simulink library "Teleop_lib"  (R2023b)
settings: Solver=VariableStepAuto  StartTime=0.0  StopTime=10.0  RelTol=1e-3
settings Model: Creator=FIRSTMentor  LastModifiedBy=ander

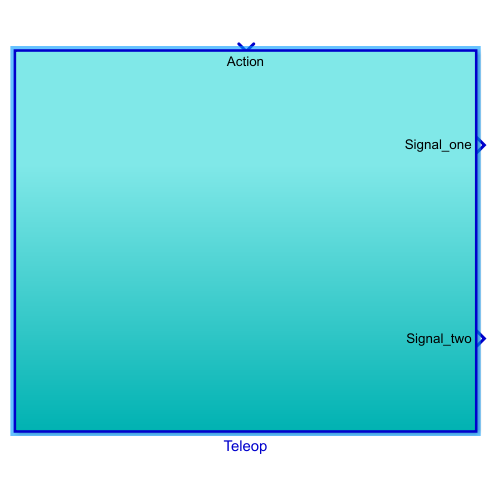
[thumbnail: Simulink's stored preview of the top-level diagram]
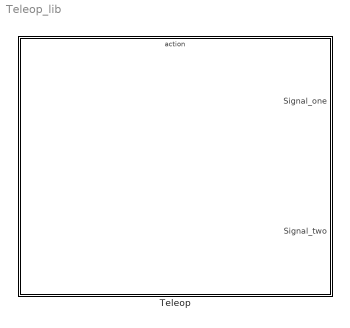
== system Teleop_lib ==
  Teleop : Subsystem  TreatAsAtomicUnit=on

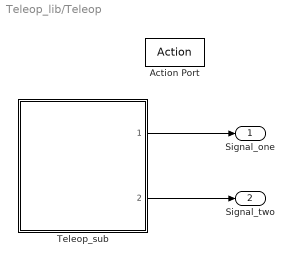
== system Teleop_lib/Teleop ==
  Action Port : ActionPort  InitializeStates=reset
  Teleop_sub : Subsystem  ReferencedSubsystem=Teleop_sub
  Signal_one : Outport
  Signal_two : Outport  Port=2
  wires:
  Teleop_sub/1 -> Signal_one/1
  Teleop_sub/2 -> Signal_two/1
